simulink model "parte4_eje1_Thidraulica_ctrl"  (R2019b)
settings: Solver=VariableStepAuto  StartTime=0.0  StopTime=20  RelTol=1e-3
settings Model: Creator=cjuar  LastModifiedBy=cjuar
settings DataIOCC: ReturnWorkspaceOutputs=off
settings DebuggingCC: ArithmeticOperatorsInVariantConditions=warning
settings SFSimCC: SimUseLocalCustomCode=off  CustomCodeUndefinedFunction=UseInterfaceOnly
settings RTWCC: RTWUseLocalCustomCode=off

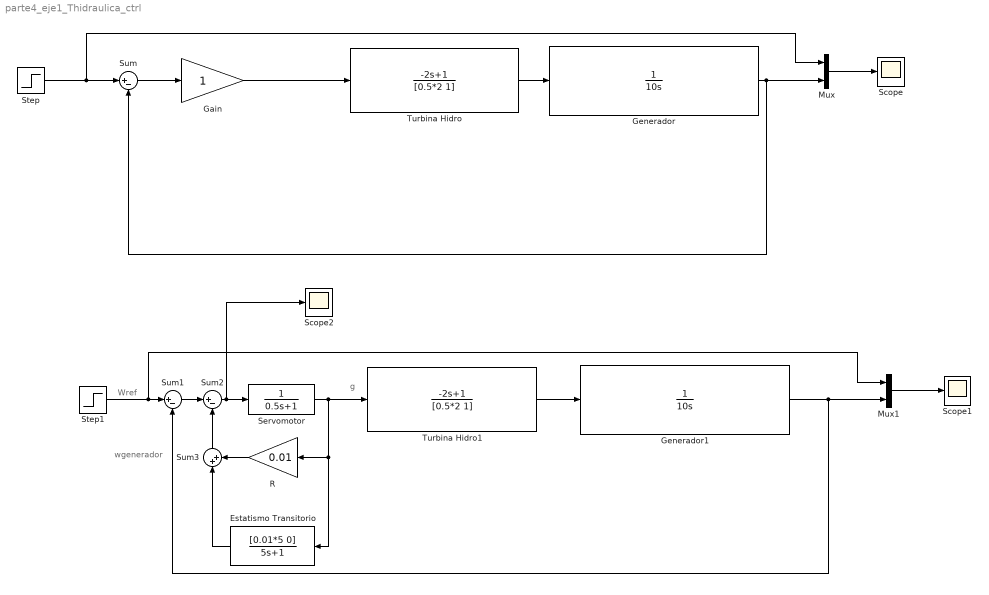
== system parte4_eje1_Thidraulica_ctrl ==
  note: g
  note: wgenerador
  note: Wref
  Estatismo Transitorio : TransferFcn  Numerator=[0.01*5 0]  Denominator=[5 1]
  Gain : Gain
  Generador : TransferFcn  Denominator=[10 0]
  Generador1 : TransferFcn  Denominator=[10 0]
  Mux : Mux  Inputs=2
  Mux1 : Mux  Inputs=2
  R : Gain  Gain=0.01
  Scope : Scope
  Scope1 : Scope
  Scope2 : Scope
  Servomotor : TransferFcn  Denominator=[0.5 1]
  Step : Step  After=0.1  SampleTime=0
  Step1 : Step  After=0.1  SampleTime=0
  Sum : Sum  Inputs=|+-
  Sum1 : Sum  Inputs=|+-
  Sum2 : Sum  Inputs=|+-
  Sum3 : Sum  Inputs=|++
  Turbina Hidro : TransferFcn  Numerator=[-2 1]  Denominator=[0.5*2 1]
  Turbina Hidro1 : TransferFcn  Numerator=[-2 1]  Denominator=[0.5*2 1]
  wires:
  Mux/1 -> Scope/1
  Turbina Hidro/1 -> Generador/1
  Gain/1 -> Turbina Hidro/1
  Sum/1 -> Gain/1
  Generador/1 -> Sum/2, Mux/2
  Step/1 -> Mux/1, Sum/1
  Step1/1 -> Mux1/1, Sum1/1
  Mux1/1 -> Scope1/1
  Sum1/1 -> Sum2/1
  Generador1/1 -> Sum1/2, Mux1/2
  Turbina Hidro1/1 -> Generador1/1
  Sum3/1 -> Sum2/2
  R/1 -> Sum3/2
  Servomotor/1 -> Estatismo Transitorio/1, R/1, Turbina Hidro1/1
  Sum2/1 -> Scope2/1, Servomotor/1
  Estatismo Transitorio/1 -> Sum3/1
